simulink library "carnotUIBK_bus"  (R2023b)
settings: Solver=VariableStepAuto  StartTime=0.0  StopTime=10.0  RelTol=1e-3  EnableMultiTasking=on
values from neighbouring files (symbols this model uses):
  A = 7*10*2    (= 140)    [theta_ground_v1.m]    (also in xlswrite1.m = num2cell(data))
  amb_factor = 1    [DOOR.m]    (also in WALL.m; WINDOW.m = 0)
  area = obj.width * obj.height    [DOOR.m]    (also in RES.m = []; ROOM.m = 0; THERMALZONE.m = area + room(kk).area; WALL.m = area - obj.doors(jj).calc_area())
  B = A/(0.5 * P)    (= 8.23529411765)    [theta_ground_v1.m]
  boundary = BOUNDARY()    [BUILDING.m]    (also in WALL.m = '')
  building = obj    [BUILDING.m]    (also in create_building_automatic.m = building.save(); ini_building_automatic.m = building.add_variant_hvac(building.variant_hvac, hvac); load_building_automatic.m = building.save())
  C = zeros(1,length(d)+1)    [CONSTRUCTION.m]    (also in DOOR.m = [0 0 0]; WALL.m = [0 0 0]; WINDOW.m = [0 0 0])
  control = 2    [GAIN.m]    (also in GAINS.m)
  cp = str2num(value)    [CONSTRUCTION.m]
  height = 0    [DOOR.m]    (also in ROOM.m; THERMALZONE.m; WALL.m; WINDOW.m)
  p = [timevec_weather weather(:,12)]    [BOUNDARY.m]    (also in WEATHER.m = 0; init_carnotUIBK.m = cell2mat(carnotUIBKpaths(i,2)))
  rho = str2num(value)    [CONSTRUCTION.m]    (also in theta_ground_v1.m = 2000)
  type = 1    [CONSTRUCTION.m]    (also in GAINS.m = raw_moisture{ii,3}; STRUCTURE.m = 0)
  view_factor = 1    [DOOR.m]    (also in WINDOW.m = 0)
  wall = []    [ROOM.m]
  z = obj.Z    [WALL.m]    (also in theta_ground_v1.m = 0)
  zone = obj.zone(ind)    [THERMALZONE.m]
undefined symbols (not defined in the file or in its folder): const, Dd, get_building, mdot_air, mdot_CO2, mdot_H2O, mdot_VOC, pos, Qdot_C, Qdot_H, Qdot_I_electricity, Qdot_I_light, Qdot_I_person, Qdot_S, Qdot_T_ground, Qdot_T_internal, Qdot_T_neighbour, Qdot_T_opaque, Qdot_T_window, Qdot_V_infiltration, Qdot_V_mech, Qdot_V_window, Qdotc, Qdotr, r_frame, solar_ratio, solar_ratio1, solar_ratio2, Tc, Tr, Ts, Uvalue, wallsurface, window, window_height, window_heigth, window_width, windowsurface, x_CO2, x_H2O, x_VOC
libraries: $bdroot x134, carnot x87, simulink_extras x14, slpidlib x4, simulink x3
(part 6 of 12)

== system carnotUIBK_bus/room_node/1-node/mass blalance ==
  mdot_H2O : Inport
  mdot_CO2 : Inport  Port=2
  mdot_VOC : Inport  Port=3
  AIB : Inport  Port=4
  (1/m^3) : Constant  Value=1/zoneairvolume
  Bus Selector1 : BusSelector  OutputSignals=rho
  m_CO2 : Integrator  InitialCondition=zonestartCO2  LimitOutput=on  LowerSaturationLimit=0
  m_H2O : Integrator  InitialCondition=zonestartWATER  LimitOutput=on  LowerSaturationLimit=0
  m_VOC : Integrator  InitialCondition=zonestartVOC  LimitOutput=on  LowerSaturationLimit=0
  x1 : Product  Inputs=**  InputSameDT=on  SaturateOnIntegerOverflow=on  OutDataTypeStr=Inherit: Same as first input
  x2 : Product  Inputs=**  InputSameDT=on  SaturateOnIntegerOverflow=on  OutDataTypeStr=Inherit: Same as first input
  x3 : Product  Inputs=**  InputSameDT=on  SaturateOnIntegerOverflow=on  OutDataTypeStr=Inherit: Same as first input
  x4 : Product  Inputs=*/  InputSameDT=on  SaturateOnIntegerOverflow=on  OutDataTypeStr=Inherit: Same as first input
  x_H2O : Outport  VectorParamsAs1DForOutWhenUnconnected=off
  x_CO2 : Outport  Port=2  VectorParamsAs1DForOutWhenUnconnected=off
  x_VOC : Outport  Port=3  VectorParamsAs1DForOutWhenUnconnected=off
  wires:
  Bus Selector1/1 -> x4/2  "<rho>"
  AIB/1 -> Bus Selector1/1
  mdot_VOC/1 -> m_VOC/1
  m_CO2/1 -> x2/1
  m_VOC/1 -> x3/1
  x4/1 -> x3/2, x2/2, x1/2
  m_H2O/1 -> x1/1
  x3/1 -> x_VOC/1  "x_VOC"
  (1/m^3)/1 -> x4/1
  x2/1 -> x_CO2/1  "x_CO2"
  x1/1 -> x_H2O/1  "x_H2O"
  mdot_H2O/1 -> m_H2O/1
  mdot_CO2/1 -> m_CO2/1

== system carnotUIBK_bus/room_node/1-node/pressure ==
  mdot_air : Inport
  AIB : Inport  Port=2
  (1/m^3) : Constant  Value=1/zoneairvolume
  Bus Selector1 : BusSelector  OutputSignals=Tc
  Subsystem : Subsystem
  Transfer Fcn (with initial outputs)1 : Subsystem  mask(Transfer Function with Initial Outputs){N=[1], D=[timeconst  1], Y0=zonestartP0, U0=1}
      mask prompts: N "Numerator:"; D "Denominator:"; Y0 "Initial output:"; U0 "Initial input:"
      mask help: Vector expressions for numerator, and denominator. Coefficients are in descending powers of s.
      mask init:
      | [A,B,C,Dd]=tf2ss(N,D);if (isempty(Y0));[m,n]=size(A);X0=zeros(1,m); end; if (isempty(U0));[m,p]=size(B);U0=zeros(1,p);end;X0=getxo(A,B,C,Dd,U0,Y0,0);
      mask Help: Specify the initial output for the transfer function.  An optimization routine attempts to determine the appropriate initial states so that the specified initial output is achieved.  For more details, see the m-file getxo.m
      mask Display: dpoly(N,D,'s')
  m_air : Integrator  InitialCondition=zonestartAIR  LimitOutput=on  LowerSaturationLimit=0
  x : Product  Inputs=***  InputSameDT=on  SaturateOnIntegerOverflow=on  OutDataTypeStr=Inherit: Same as first input
  p : Outport  VectorParamsAs1DForOutWhenUnconnected=off
  wires:
  Transfer Fcn (with initial outputs)1/1(Out1) -> p/1  "p"
  Subsystem/1(R*T ') -> x/2
  (1/m^3)/1 -> x/3
  m_air/1 -> x/1
  AIB/1 -> Bus Selector1/1
  Bus Selector1/1 -> Subsystem/1(T)  "<Tc>"
  x/1 -> Transfer Fcn (with initial outputs)1/1(In1)
  mdot_air/1 -> m_air/1

== system carnotUIBK_bus/room_node/1-node/sensitive_node ==
  note: SENSITIVE node
  Qdotc : Inport
  Qdotr : Inport  Port=2
  Add : Sum
  Integrator : Integrator  InitialCondition=zonestartTEMP
  mcp : Constant  Value=1/mcp
  x3 : Product  Inputs=**  InputSameDT=on  SaturateOnIntegerOverflow=on  OutDataTypeStr=Inherit: Same as first input
  Tc : Outport  VectorParamsAs1DForOutWhenUnconnected=off
  wires:
  x3/1 -> Integrator/1
  Integrator/1 -> Tc/1
  Add/1 -> x3/1
  Qdotc/1 -> Add/2
  Qdotr/1 -> Add/1
  mcp/1 -> x3/2

== system carnotUIBK_bus/room_node/1-node_womass/sensitive_node ==
  note: SENSITIVE node
  Qdotc : Inport
  Qdotr : Inport  Port=2
  Add : Sum
  Integrator : Integrator  InitialCondition=zonestartTEMP
  mcp : Constant  Value=1/mcp
  x3 : Product  Inputs=**  InputSameDT=on  SaturateOnIntegerOverflow=on  OutDataTypeStr=Inherit: Same as first input
  Tc : Outport  VectorParamsAs1DForOutWhenUnconnected=off
  wires:
  x3/1 -> Integrator/1
  Integrator/1 -> Tc/1
  Add/1 -> x3/1
  Qdotc/1 -> Add/2
  Qdotr/1 -> Add/1
  mcp/1 -> x3/2

== system carnotUIBK_bus/room_node/2-node/Sensitive room temperature ==
  note: Sensitive temperature
  Tr : Inport
  Tc : Inport  Port=2
  1-share_c : Gain  Gain=1-share_c  SaturateOnIntegerOverflow=on  OutDataTypeStr=Inherit: Same as input  ParamDataTypeStr=Inherit: Same as input
  Sum : Sum  InputSameDT=on  SaturateOnIntegerOverflow=on  OutDataTypeStr=Inherit: Same as first input
  share_c : Gain  Gain=share_c  SaturateOnIntegerOverflow=on  OutDataTypeStr=Inherit: Same as input  ParamDataTypeStr=Inherit: Same as input
  Ts : Outport  VectorParamsAs1DForOutWhenUnconnected=off
  wires:
  Tr/1 -> 1-share_c/1
  Tc/1 -> share_c/1
  share_c/1 -> Sum/1  "Tc"
  1-share_c/1 -> Sum/2  "Tr"
  Sum/1 -> Ts/1

== system carnotUIBK_bus/room_node/2-node/convective_node ==
  note: CONVECTIVE node
  Qdotc : Inport
  AIB : Inport  Port=2
  (1/m^3) : Constant  Value=1/zoneairvolume
  Bus Selector1 : BusSelector  OutputSignals=rho,cp
  Integrator : Integrator  InitialCondition=zonestartTEMP
  x3 : Product  Inputs=**  InputSameDT=on  SaturateOnIntegerOverflow=on  OutDataTypeStr=Inherit: Same as first input
  x4 : Product  Inputs=*//  InputSameDT=on  SaturateOnIntegerOverflow=on  OutDataTypeStr=Inherit: Same as first input
  Tc : Outport  VectorParamsAs1DForOutWhenUnconnected=off
  wires:
  Bus Selector1/2 -> x4/3  "<cp>"
  Bus Selector1/1 -> x4/2  "<rho>"
  AIB/1 -> Bus Selector1/1
  x3/1 -> Integrator/1
  (1/m^3)/1 -> x4/1
  x4/1 -> x3/2
  Integrator/1 -> Tc/1
  Qdotc/1 -> x3/1

== system carnotUIBK_bus/room_node/2-node/density and capacity ==
  T : Inport
  p : Inport  Port=2
  fluid_type : Inport  Port=3
  fluid_mix : Inport  Port=4
  Add : Sum  Inputs=2
  Constant1 : Constant  Value=10000
  Constant2 : Constant  Value=0.0001
  Divide : Product  Inputs=*/
  K : Constant  Value=273.15
  Product : Product
  Product1 : Product
  Ra : Gain  Gain=287.058
  Rounding Function : Rounding
  Terminator : Terminator
  Terminator1 : Terminator
  Transfer Fcn (with initial outputs) : Subsystem  mask(Transfer Function with Initial Outputs){N=[1], D=[timeconst  1], Y0=1.1893, U0=1}
      mask prompts: N "Numerator:"; D "Denominator:"; Y0 "Initial output:"; U0 "Initial input:"
      mask help: Vector expressions for numerator, and denominator. Coefficients are in descending powers of s.
      mask init:
      | [A,B,C,Dd]=tf2ss(N,D);if (isempty(Y0));[m,n]=size(A);X0=zeros(1,m); end; if (isempty(U0));[m,p]=size(B);U0=zeros(1,p);end;X0=getxo(A,B,C,Dd,U0,Y0,0);
      mask Help: Specify the initial output for the transfer function.  An optimization routine attempts to determine the appropriate initial states so that the specified initial output is achieved.  For more details, see the m-file getxo.m
      mask Display: dpoly(N,D,'s')
  cp_const : Constant  Value=1006.8
  rho : Outport  VectorParamsAs1DForOutWhenUnconnected=off
  cp : Outport  Port=2  VectorParamsAs1DForOutWhenUnconnected=off
  wires:
  cp_const/1 -> cp/1
  Divide/1 -> Transfer Fcn (with initial outputs)/1(In1)
  p/1 -> Divide/1
  fluid_type/1 -> Terminator/1
  fluid_mix/1 -> Terminator1/1
  T/1 -> Add/1
  K/1 -> Add/2
  Add/1 -> Ra/1
  Ra/1 -> Divide/2
  Rounding Function/1 -> Product1/1
  Transfer Fcn (with initial outputs)/1(Out1) -> Product/1
  Product/1 -> Rounding Function/1
  Constant1/1 -> Product/2
  Constant2/1 -> Product1/2
  Product1/1 -> rho/1

== system carnotUIBK_bus/room_node/2-node/mass blalance ==
  mdot_H2O : Inport
  mdot_CO2 : Inport  Port=2
  mdot_VOC : Inport  Port=3
  AIB : Inport  Port=4
  (1/m^3) : Constant  Value=1/zoneairvolume
  Bus Selector1 : BusSelector  OutputSignals=rho
  m_CO2 : Integrator  InitialCondition=zonestartCO2  LimitOutput=on  LowerSaturationLimit=0
  m_H2O : Integrator  InitialCondition=zonestartWATER  LimitOutput=on  LowerSaturationLimit=0
  m_VOC : Integrator  InitialCondition=zonestartVOC  LimitOutput=on  LowerSaturationLimit=0
  x1 : Product  Inputs=**  InputSameDT=on  SaturateOnIntegerOverflow=on  OutDataTypeStr=Inherit: Same as first input
  x2 : Product  Inputs=**  InputSameDT=on  SaturateOnIntegerOverflow=on  OutDataTypeStr=Inherit: Same as first input
  x3 : Product  Inputs=**  InputSameDT=on  SaturateOnIntegerOverflow=on  OutDataTypeStr=Inherit: Same as first input
  x4 : Product  Inputs=*/  InputSameDT=on  SaturateOnIntegerOverflow=on  OutDataTypeStr=Inherit: Same as first input
  x_H2O : Outport  VectorParamsAs1DForOutWhenUnconnected=off
  x_CO2 : Outport  Port=2  VectorParamsAs1DForOutWhenUnconnected=off
  x_VOC : Outport  Port=3  VectorParamsAs1DForOutWhenUnconnected=off
  wires:
  Bus Selector1/1 -> x4/2  "<rho>"
  AIB/1 -> Bus Selector1/1
  mdot_VOC/1 -> m_VOC/1
  m_CO2/1 -> x2/1
  m_VOC/1 -> x3/1
  x4/1 -> x3/2, x2/2, x1/2
  m_H2O/1 -> x1/1
  x3/1 -> x_VOC/1  "x_VOC"
  (1/m^3)/1 -> x4/1
  x2/1 -> x_CO2/1  "x_CO2"
  x1/1 -> x_H2O/1  "x_H2O"
  mdot_H2O/1 -> m_H2O/1
  mdot_CO2/1 -> m_CO2/1

== system carnotUIBK_bus/room_node/2-node/pressure ==
  mdot_air : Inport
  AIB : Inport  Port=2
  (1/m^3) : Constant  Commented=on  Value=1/zoneairvolume
  Bus Selector1 : BusSelector  Commented=on  OutputSignals=Tc
  Subsystem : Subsystem  Commented=on
  Transfer Fcn (with initial outputs)1 : Subsystem  Commented=on  mask(Transfer Function with Initial Outputs){N=[1], D=[timeconst  1], Y0=zonestartP0, U0=1}
      mask prompts: N "Numerator:"; D "Denominator:"; Y0 "Initial output:"; U0 "Initial input:"
      mask help: Vector expressions for numerator, and denominator. Coefficients are in descending powers of s.
      mask init:
      | [A,B,C,Dd]=tf2ss(N,D);if (isempty(Y0));[m,n]=size(A);X0=zeros(1,m); end; if (isempty(U0));[m,p]=size(B);U0=zeros(1,p);end;X0=getxo(A,B,C,Dd,U0,Y0,0);
      mask Help: Specify the initial output for the transfer function.  An optimization routine attempts to determine the appropriate initial states so that the specified initial output is achieved.  For more details, see the m-file getxo.m
      mask Display: dpoly(N,D,'s')
  convert2U32 : DataTypeConversion  Commented=on  OutDataTypeStr=uint32  SaturateOnIntegerOverflow=off  RndMeth=Floor
  convert2double : DataTypeConversion  Commented=on  OutDataTypeStr=double  SaturateOnIntegerOverflow=off  RndMeth=Floor
  m_air : Integrator  Commented=on  InitialCondition=zonestartAIR  LimitOutput=on  LowerSaturationLimit=0
  p0 : Constant  Value=1e5
  x : Product  Commented=on  Inputs=***  InputSameDT=on  SaturateOnIntegerOverflow=on  OutDataTypeStr=Inherit: Same as first input
  p : Outport  VectorParamsAs1DForOutWhenUnconnected=off
  wires:
  Transfer Fcn (with initial outputs)1/1(Out1) -> convert2U32/1  "p"
  Subsystem/1(R*T ') -> x/2
  (1/m^3)/1 -> x/3
  m_air/1 -> x/1
  AIB/1 -> Bus Selector1/1
  Bus Selector1/1 -> Subsystem/1(T)  "<Tc>"
  x/1 -> Transfer Fcn (with initial outputs)1/1(In1)
  mdot_air/1 -> m_air/1
  convert2U32/1 -> convert2double/1
  p0/1 -> p/1

== system carnotUIBK_bus/room_node/2-node/radiative_node ==
  note: RADIATIVE node
  Qdotr : Inport
  Gain : Gain  Gain=1/timeconst
  Integrator : Integrator  InitialCondition=zonestartTEMP
  Tr : Outport  VectorParamsAs1DForOutWhenUnconnected=off
  wires:
  Integrator/1 -> Tr/1
  Qdotr/1 -> Gain/1
  Gain/1 -> Integrator/1

== system carnotUIBK_bus/room_node/2-node_ideal/Sensitive room temperature ==
  note: Sensitive temperature
  Tr : Inport
  Tc : Inport  Port=2
  1-share_c : Gain  Gain=1-share_c  SaturateOnIntegerOverflow=on  OutDataTypeStr=Inherit: Same as input  ParamDataTypeStr=Inherit: Same as input
  Sum : Sum  InputSameDT=on  SaturateOnIntegerOverflow=on  OutDataTypeStr=Inherit: Same as first input
  share_c : Gain  Gain=share_c  SaturateOnIntegerOverflow=on  OutDataTypeStr=Inherit: Same as input  ParamDataTypeStr=Inherit: Same as input
  Ts : Outport  VectorParamsAs1DForOutWhenUnconnected=off
  wires:
  Tr/1 -> 1-share_c/1
  Tc/1 -> share_c/1
  share_c/1 -> Sum/1  "Tc"
  1-share_c/1 -> Sum/2  "Tr"
  Sum/1 -> Ts/1

== system carnotUIBK_bus/room_node/2-node_ideal/mass blalance ==
  mdot_H2O : Inport
  mdot_CO2 : Inport  Port=2
  mdot_VOC : Inport  Port=3
  AIB : Inport  Port=4
  (1/m^3) : Constant  Value=1/zoneairvolume
  Bus Selector1 : BusSelector  OutputSignals=rho
  m_CO2 : Integrator  InitialCondition=zonestartCO2  LimitOutput=on  LowerSaturationLimit=0
  m_H2O : Integrator  InitialCondition=zonestartWATER  LimitOutput=on  LowerSaturationLimit=0
  m_VOC : Integrator  InitialCondition=zonestartVOC  LimitOutput=on  LowerSaturationLimit=0
  x1 : Product  Inputs=**  InputSameDT=on  SaturateOnIntegerOverflow=on  OutDataTypeStr=Inherit: Same as first input
  x2 : Product  Inputs=**  InputSameDT=on  SaturateOnIntegerOverflow=on  OutDataTypeStr=Inherit: Same as first input
  x3 : Product  Inputs=**  InputSameDT=on  SaturateOnIntegerOverflow=on  OutDataTypeStr=Inherit: Same as first input
  x4 : Product  Inputs=*/  InputSameDT=on  SaturateOnIntegerOverflow=on  OutDataTypeStr=Inherit: Same as first input
  x_H2O : Outport  VectorParamsAs1DForOutWhenUnconnected=off
  x_CO2 : Outport  Port=2  VectorParamsAs1DForOutWhenUnconnected=off
  x_VOC : Outport  Port=3  VectorParamsAs1DForOutWhenUnconnected=off
  wires:
  Bus Selector1/1 -> x4/2  "<rho>"
  AIB/1 -> Bus Selector1/1
  mdot_VOC/1 -> m_VOC/1
  m_CO2/1 -> x2/1
  m_VOC/1 -> x3/1
  x4/1 -> x3/2, x2/2, x1/2
  m_H2O/1 -> x1/1
  x3/1 -> x_VOC/1  "x_VOC"
  (1/m^3)/1 -> x4/1
  x2/1 -> x_CO2/1  "x_CO2"
  x1/1 -> x_H2O/1  "x_H2O"
  mdot_H2O/1 -> m_H2O/1
  mdot_CO2/1 -> m_CO2/1

== system carnotUIBK_bus/room_node/2-node_ideal/pressure ==
  mdot_air : Inport
  AIB : Inport  Port=2
  (1/m^3) : Constant  Value=1/zoneairvolume
  Bus Selector1 : BusSelector  OutputSignals=Tc
  Subsystem : Subsystem
  Transfer Fcn (with initial outputs)1 : Subsystem  mask(Transfer Function with Initial Outputs){N=[1], D=[timeconst  1], Y0=zonestartP0, U0=1}
      mask prompts: N "Numerator:"; D "Denominator:"; Y0 "Initial output:"; U0 "Initial input:"
      mask help: Vector expressions for numerator, and denominator. Coefficients are in descending powers of s.
      mask init:
      | [A,B,C,Dd]=tf2ss(N,D);if (isempty(Y0));[m,n]=size(A);X0=zeros(1,m); end; if (isempty(U0));[m,p]=size(B);U0=zeros(1,p);end;X0=getxo(A,B,C,Dd,U0,Y0,0);
      mask Help: Specify the initial output for the transfer function.  An optimization routine attempts to determine the appropriate initial states so that the specified initial output is achieved.  For more details, see the m-file getxo.m
      mask Display: dpoly(N,D,'s')
  m_air : Integrator  InitialCondition=zonestartAIR  LimitOutput=on  LowerSaturationLimit=0
  x : Product  Inputs=***  InputSameDT=on  SaturateOnIntegerOverflow=on  OutDataTypeStr=Inherit: Same as first input
  p : Outport  VectorParamsAs1DForOutWhenUnconnected=off
  wires:
  Transfer Fcn (with initial outputs)1/1(Out1) -> p/1  "p"
  Subsystem/1(R*T ') -> x/2
  (1/m^3)/1 -> x/3
  m_air/1 -> x/1
  AIB/1 -> Bus Selector1/1
  Bus Selector1/1 -> Subsystem/1(T)  "<Tc>"
  x/1 -> Transfer Fcn (with initial outputs)1/1(In1)
  mdot_air/1 -> m_air/1

== system carnotUIBK_bus/room_node/EMPTY/AIB_initialize ==
  Bus Creator2 : BusCreator  Inputs=9
  Constant{,1..8} (9 alike) : Constant  Value=0
  AIB : Outport  VectorParamsAs1DForOutWhenUnconnected=off
  wires:
  Bus Creator2/1 -> AIB/1
  Constant4/1 -> Bus Creator2/5  "x_CO2"
  Constant2/1 -> Bus Creator2/3  "Tr"
  Constant1/1 -> Bus Creator2/2  "Tc"
  Constant6/1 -> Bus Creator2/7  "rho"
  Constant7/1 -> Bus Creator2/8  "cp"
  Constant/1 -> Bus Creator2/1  "Ts"
  Constant8/1 -> Bus Creator2/9  "p"
  Constant3/1 -> Bus Creator2/4  "x_H2O"
  Constant5/1 -> Bus Creator2/6  "x_VOC"

== system carnotUIBK_bus/room_node/EMPTY/Sensitive room temperature ==
  note: Sensitive temperature
  Tr : Inport
  Tc : Inport  Port=2
  1-share_c : Gain  Gain=1-share_c  SaturateOnIntegerOverflow=on  OutDataTypeStr=Inherit: Same as input  ParamDataTypeStr=Inherit: Same as input
  Sum : Sum  InputSameDT=on  SaturateOnIntegerOverflow=on  OutDataTypeStr=Inherit: Same as first input
  share_c : Gain  Gain=share_c  SaturateOnIntegerOverflow=on  OutDataTypeStr=Inherit: Same as input  ParamDataTypeStr=Inherit: Same as input
  Ts : Outport  VectorParamsAs1DForOutWhenUnconnected=off
  wires:
  Tr/1 -> 1-share_c/1
  Tc/1 -> share_c/1
  share_c/1 -> Sum/1  "Tc"
  1-share_c/1 -> Sum/2  "Tr"
  Sum/1 -> Ts/1

== system carnotUIBK_bus/wall_intersection/R-C model/alpha_i1 ==
  Ts : Inport
  AIB : Inport  Port=2
  Qdot sol : Inport  Port=3
  phis : Inport  Port=4
  alpha_i_down : Subsystem  VariantControl=V_i_XXX_XXX_wXXX_hti2  mask(ALFA){}
      mask help:
      | Convective and radiative heat transfer at the INDOOR SURFACE of a VERTICAL OUTER WALL.
      |
      | [AIV] : conditions of zone node,
      | Ts : temperature of wall surface, °C,
      | qdots : specific heat flow into wall construction, W/m^2,
      | [S] : heat and air flow to zone node.
  alpha_i_horizontal : Subsystem  VariantControl=V_i_XXX_XXX_wXXX_hti0  mask(ALFA){}
      mask help:
      | Convective and radiative heat transfer at the INDOOR SURFACE of a VERTICAL OUTER WALL.
      |
      | [AIV] : conditions of zone node,
      | Ts : temperature of wall surface, °C,
      | qdots : specific heat flow into wall construction, W/m^2,
      | [S] : heat and air flow to zone node.
  alpha_i_up : Subsystem  VariantControl=V_i_XXX_XXX_wXXX_hti1  mask(ALFA){}
      mask help:
      | Convective and radiative heat transfer at the INDOOR SURFACE of a VERTICAL OUTER WALL.
      |
      | [AIV] : conditions of zone node,
      | Ts : temperature of wall surface, °C,
      | qdots : specific heat flow into wall construction, W/m^2,
      | [S] : heat and air flow to zone node.
  qdots : Outport  VectorParamsAs1DForOutWhenUnconnected=off
  "[S]" : Outport  Port=2  VectorParamsAs1DForOutWhenUnconnected=off
  alpha_c : Outport  Port=3  VectorParamsAs1DForOutWhenUnconnected=off
  phi_i_1/100 : Outport  Port=4  VectorParamsAs1DForOutWhenUnconnected=off

== system carnotUIBK_bus/wall_intersection/R-C model/alpha_i2 ==
  Ts : Inport
  AIB : Inport  Port=2
  Qdot sol : Inport  Port=3
  phis : Inport  Port=4
  alpha_i_down : Subsystem  VariantControl=V_i_XXX_XXX_wXXX_hti2  mask(ALFA){}
      mask help:
      | Convective and radiative heat transfer at the INDOOR SURFACE of a VERTICAL OUTER WALL.
      |
      | [AIV] : conditions of zone node,
      | Ts : temperature of wall surface, °C,
      | qdots : specific heat flow into wall construction, W/m^2,
      | [S] : heat and air flow to zone node.
  alpha_i_horizontal : Subsystem  VariantControl=V_i_XXX_XXX_wXXX_hti0  mask(ALFA){}
      mask help:
      | Convective and radiative heat transfer at the INDOOR SURFACE of a VERTICAL OUTER WALL.
      |
      | [AIV] : conditions of zone node,
      | Ts : temperature of wall surface, °C,
      | qdots : specific heat flow into wall construction, W/m^2,
      | [S] : heat and air flow to zone node.
  alpha_i_up : Subsystem  VariantControl=V_i_XXX_XXX_wXXX_hti1  mask(ALFA){}
      mask help:
      | Convective and radiative heat transfer at the INDOOR SURFACE of a VERTICAL OUTER WALL.
      |
      | [AIV] : conditions of zone node,
      | Ts : temperature of wall surface, °C,
      | qdots : specific heat flow into wall construction, W/m^2,
      | [S] : heat and air flow to zone node.
  qdots : Outport  VectorParamsAs1DForOutWhenUnconnected=off
  "[S]" : Outport  Port=2  VectorParamsAs1DForOutWhenUnconnected=off
  alpha_c : Outport  Port=3  VectorParamsAs1DForOutWhenUnconnected=off
  phi_i_1/100 : Outport  Port=4  VectorParamsAs1DForOutWhenUnconnected=off

== system carnotUIBK_bus/wall_intersection/UA/Rsi ==
  down : Subsystem  VariantControl=V_i_XXX_XXX_wXXX_hti2
  horizontal : Subsystem  VariantControl=V_i_XXX_XXX_wXXX_hti0
  up : Subsystem  VariantControl=V_i_XXX_XXX_wXXX_hti1
  Rsi : Outport  VectorParamsAs1DForOutWhenUnconnected=off

== system carnotUIBK_bus/wall_intersection/hygrothermal model/alpha_i1 ==
  Ts : Inport
  AIB : Inport  Port=2
  Qdot sol : Inport  Port=3
  phis : Inport  Port=4
  alpha_i_down : Subsystem  VariantControl=V_i_XXX_XXX_wXXX_hti2  mask(ALFA){}
      mask help:
      | Convective and radiative heat transfer at the INDOOR SURFACE of a VERTICAL OUTER WALL.
      |
      | [AIV] : conditions of zone node,
      | Ts : temperature of wall surface, °C,
      | qdots : specific heat flow into wall construction, W/m^2,
      | [S] : heat and air flow to zone node.
  alpha_i_horizontal : Subsystem  VariantControl=V_i_XXX_XXX_wXXX_hti0  mask(ALFA){}
      mask help:
      | Convective and radiative heat transfer at the INDOOR SURFACE of a VERTICAL OUTER WALL.
      |
      | [AIV] : conditions of zone node,
      | Ts : temperature of wall surface, °C,
      | qdots : specific heat flow into wall construction, W/m^2,
      | [S] : heat and air flow to zone node.
  alpha_i_up : Subsystem  VariantControl=V_i_XXX_XXX_wXXX_hti1  mask(ALFA){}
      mask help:
      | Convective and radiative heat transfer at the INDOOR SURFACE of a VERTICAL OUTER WALL.
      |
      | [AIV] : conditions of zone node,
      | Ts : temperature of wall surface, °C,
      | qdots : specific heat flow into wall construction, W/m^2,
      | [S] : heat and air flow to zone node.
  qdots : Outport  VectorParamsAs1DForOutWhenUnconnected=off
  "[S]" : Outport  Port=2  VectorParamsAs1DForOutWhenUnconnected=off
  alpha_c : Outport  Port=3  VectorParamsAs1DForOutWhenUnconnected=off
  phi_i_1/100 : Outport  Port=4  VectorParamsAs1DForOutWhenUnconnected=off

== system carnotUIBK_bus/wall_intersection/hygrothermal model/alpha_i2 ==
  Ts : Inport
  AIB : Inport  Port=2
  Qdot sol : Inport  Port=3
  phis : Inport  Port=4
  alpha_i_down : Subsystem  VariantControl=V_i_XXX_XXX_wXXX_hti2  mask(ALFA){}
      mask help:
      | Convective and radiative heat transfer at the INDOOR SURFACE of a VERTICAL OUTER WALL.
      |
      | [AIV] : conditions of zone node,
      | Ts : temperature of wall surface, °C,
      | qdots : specific heat flow into wall construction, W/m^2,
      | [S] : heat and air flow to zone node.
  alpha_i_horizontal : Subsystem  VariantControl=V_i_XXX_XXX_wXXX_hti0  mask(ALFA){}
      mask help:
      | Convective and radiative heat transfer at the INDOOR SURFACE of a VERTICAL OUTER WALL.
      |
      | [AIV] : conditions of zone node,
      | Ts : temperature of wall surface, °C,
      | qdots : specific heat flow into wall construction, W/m^2,
      | [S] : heat and air flow to zone node.
  alpha_i_up : Subsystem  VariantControl=V_i_XXX_XXX_wXXX_hti1  mask(ALFA){}
      mask help:
      | Convective and radiative heat transfer at the INDOOR SURFACE of a VERTICAL OUTER WALL.
      |
      | [AIV] : conditions of zone node,
      | Ts : temperature of wall surface, °C,
      | qdots : specific heat flow into wall construction, W/m^2,
      | [S] : heat and air flow to zone node.
  qdots : Outport  VectorParamsAs1DForOutWhenUnconnected=off
  "[S]" : Outport  Port=2  VectorParamsAs1DForOutWhenUnconnected=off
  alpha_c : Outport  Port=3  VectorParamsAs1DForOutWhenUnconnected=off
  phi_i_1/100 : Outport  Port=4  VectorParamsAs1DForOutWhenUnconnected=off

== system carnotUIBK_bus/wall_zone/R-C model/alpha_e ==
  WDB : Inport
  GDB : Inport  Port=2
  NDB : Inport  Port=3
  AIB : Inport  Port=4
  Ts : Inport  Port=5
  Qdot_sol : Inport  Port=6
  phis : Inport  Port=7
  alpha_e_AMBIENT : Subsystem  VariantControl=V_zXXX_wXXX_hte0  mask(ALFA){}
      mask help:
      | Convective and radiative HEAT TRANSFER at the WEATHER EXPOSED SURFACE of an OUTER WALL.
      |
      | [W*] : modified weather data, adapted to height over ground,
      | Ts : temperature of outdoor wall surface, °C,
      | qdots : specific heat flow into wall / window construction, W/m^2.
  alpha_e_GROUND : Subsystem  VariantControl=V_zXXX_wXXX_hte1  mask(ALFA){}
      mask help:
      | Convective and radiative HEAT TRANSFER at the WEATHER EXPOSED SURFACE of an OUTER WALL.
      |
      | [W*] : modified weather data, adapted to height over ground,
      | Ts : temperature of outdoor wall surface, °C,
      | qdots : specific heat flow into wall / window construction, W/m^2.
  alpha_e_INTERNAL : Subsystem  VariantControl=V_zXXX_wXXX_hte2  mask(ALFA){}
      mask help:
      | Convective and radiative HEAT TRANSFER at the WEATHER EXPOSED SURFACE of an OUTER WALL.
      |
      | [W*] : modified weather data, adapted to height over ground,
      | Ts : temperature of outdoor wall surface, °C,
      | qdots : specific heat flow into wall / window construction, W/m^2.
  alpha_e_NEIGHBOUR : Subsystem  VariantControl=V_zXXX_wXXX_hte3  mask(ALFA){}
      mask help:
      | Convective and radiative HEAT TRANSFER at the WEATHER EXPOSED SURFACE of an OUTER WALL.
      |
      | [W*] : modified weather data, adapted to height over ground,
      | Ts : temperature of outdoor wall surface, °C,
      | qdots : specific heat flow into wall / window construction, W/m^2.
  qdots : Outport  VectorParamsAs1DForOutWhenUnconnected=off
  "[S]" : Outport  Port=2  VectorParamsAs1DForOutWhenUnconnected=off
  alpha_c : Outport  Port=3  VectorParamsAs1DForOutWhenUnconnected=off
  phi_e_1/100 : Outport  Port=4  VectorParamsAs1DForOutWhenUnconnected=off
  theta_e : Outport  Port=5  VectorParamsAs1DForOutWhenUnconnected=off

== system carnotUIBK_bus/wall_zone/R-C model/alpha_i ==
  Ts : Inport
  AIB : Inport  Port=2
  Qdot sol : Inport  Port=3
  phis : Inport  Port=4
  alpha_i_down : Subsystem  VariantControl=V_zXXX_wXXX_hti2  mask(ALFA){}
      mask help:
      | Convective and radiative heat transfer at the INDOOR SURFACE of a VERTICAL OUTER WALL.
      |
      | [AIV] : conditions of zone node,
      | Ts : temperature of wall surface, °C,
      | qdots : specific heat flow into wall construction, W/m^2,
      | [S] : heat and air flow to zone node.
  alpha_i_horizontal : Subsystem  VariantControl=V_zXXX_wXXX_hti0  mask(ALFA){}
      mask help:
      | Convective and radiative heat transfer at the INDOOR SURFACE of a VERTICAL OUTER WALL.
      |
      | [AIV] : conditions of zone node,
      | Ts : temperature of wall surface, °C,
      | qdots : specific heat flow into wall construction, W/m^2,
      | [S] : heat and air flow to zone node.
  alpha_i_up : Subsystem  VariantControl=V_zXXX_wXXX_hti1  mask(ALFA){}
      mask help:
      | Convective and radiative heat transfer at the INDOOR SURFACE of a VERTICAL OUTER WALL.
      |
      | [AIV] : conditions of zone node,
      | Ts : temperature of wall surface, °C,
      | qdots : specific heat flow into wall construction, W/m^2,
      | [S] : heat and air flow to zone node.
  qdots : Outport  VectorParamsAs1DForOutWhenUnconnected=off
  "[S]" : Outport  Port=2  VectorParamsAs1DForOutWhenUnconnected=off
  alpha_c : Outport  Port=3  VectorParamsAs1DForOutWhenUnconnected=off
  phi_i_1/100 : Outport  Port=4  VectorParamsAs1DForOutWhenUnconnected=off

== system carnotUIBK_bus/wall_zone/UA/Rse ==
  WDB : Inport
  GDB : Inport  Port=2
  NDB : Inport  Port=3
  AIB : Inport  Port=4
  Qdot_sol : Inport  Port=5
  Qdot_in : Inport  Port=6
  R : Inport  Port=7
  Rsi : Inport  Port=8
  AMBIENT : Subsystem  VariantControl=V_zXXX_wXXX_hte0
  GROUND : Subsystem  VariantControl=V_zXXX_wXXX_hte1
  INTERNAL : Subsystem  VariantControl=V_zXXX_wXXX_hte2
  NEIGHBOUR : Subsystem  VariantControl=V_zXXX_wXXX_hte3
  "[S]" : Outport  VectorParamsAs1DForOutWhenUnconnected=off

== system carnotUIBK_bus/wall_zone/UA/Rsi ==
  down : Subsystem  VariantControl=V_zXXX_wXXX_hti2
  horizontal : Subsystem  VariantControl=V_zXXX_wXXX_hti0
  up : Subsystem  VariantControl=V_zXXX_wXXX_hti1
  Rsi : Outport  VectorParamsAs1DForOutWhenUnconnected=off

== system carnotUIBK_bus/wall_zone/hygrothermal model/alpha_e ==
  WDB : Inport
  GDB : Inport  Port=2
  NDB : Inport  Port=3
  AIB : Inport  Port=4
  Ts : Inport  Port=5
  Qdot_sol : Inport  Port=6
  phis : Inport  Port=7
  alpha_e_AMBIENT : Subsystem  VariantControl=V_zXXX_wXXX_hte0  mask(ALFA){}
      mask help:
      | Convective and radiative HEAT TRANSFER at the WEATHER EXPOSED SURFACE of an OUTER WALL.
      |
      | [W*] : modified weather data, adapted to height over ground,
      | Ts : temperature of outdoor wall surface, °C,
      | qdots : specific heat flow into wall / window construction, W/m^2.
  alpha_e_GROUND : Subsystem  VariantControl=V_zXXX_wXXX_hte1  mask(ALFA){}
      mask help:
      | Convective and radiative HEAT TRANSFER at the WEATHER EXPOSED SURFACE of an OUTER WALL.
      |
      | [W*] : modified weather data, adapted to height over ground,
      | Ts : temperature of outdoor wall surface, °C,
      | qdots : specific heat flow into wall / window construction, W/m^2.
  alpha_e_INTERNAL : Subsystem  VariantControl=V_zXXX_wXXX_hte2  mask(ALFA){}
      mask help:
      | Convective and radiative HEAT TRANSFER at the WEATHER EXPOSED SURFACE of an OUTER WALL.
      |
      | [W*] : modified weather data, adapted to height over ground,
      | Ts : temperature of outdoor wall surface, °C,
      | qdots : specific heat flow into wall / window construction, W/m^2.
  alpha_e_NEIGHBOUR : Subsystem  VariantControl=V_zXXX_wXXX_hte3  mask(ALFA){}
      mask help:
      | Convective and radiative HEAT TRANSFER at the WEATHER EXPOSED SURFACE of an OUTER WALL.
      |
      | [W*] : modified weather data, adapted to height over ground,
      | Ts : temperature of outdoor wall surface, °C,
      | qdots : specific heat flow into wall / window construction, W/m^2.
  qdots : Outport  VectorParamsAs1DForOutWhenUnconnected=off
  "[S]" : Outport  Port=2  VectorParamsAs1DForOutWhenUnconnected=off
  alpha_c : Outport  Port=3  VectorParamsAs1DForOutWhenUnconnected=off
  phi_e_1/100 : Outport  Port=4  VectorParamsAs1DForOutWhenUnconnected=off
  theta_e : Outport  Port=5  VectorParamsAs1DForOutWhenUnconnected=off

== system carnotUIBK_bus/wall_zone/hygrothermal model/alpha_i ==
  Ts : Inport
  AIB : Inport  Port=2
  Qdot sol : Inport  Port=3
  phis : Inport  Port=4
  alpha_i_down : Subsystem  VariantControl=V_zXXX_wXXX_hti2  mask(ALFA){}
      mask help:
      | Convective and radiative heat transfer at the INDOOR SURFACE of a VERTICAL OUTER WALL.
      |
      | [AIV] : conditions of zone node,
      | Ts : temperature of wall surface, °C,
      | qdots : specific heat flow into wall construction, W/m^2,
      | [S] : heat and air flow to zone node.
  alpha_i_horizontal : Subsystem  VariantControl=V_zXXX_wXXX_hti0  mask(ALFA){}
      mask help:
      | Convective and radiative heat transfer at the INDOOR SURFACE of a VERTICAL OUTER WALL.
      |
      | [AIV] : conditions of zone node,
      | Ts : temperature of wall surface, °C,
      | qdots : specific heat flow into wall construction, W/m^2,
      | [S] : heat and air flow to zone node.
  alpha_i_up : Subsystem  VariantControl=V_zXXX_wXXX_hti1  mask(ALFA){}
      mask help:
      | Convective and radiative heat transfer at the INDOOR SURFACE of a VERTICAL OUTER WALL.
      |
      | [AIV] : conditions of zone node,
      | Ts : temperature of wall surface, °C,
      | qdots : specific heat flow into wall construction, W/m^2,
      | [S] : heat and air flow to zone node.
  qdots : Outport  VectorParamsAs1DForOutWhenUnconnected=off
  "[S]" : Outport  Port=2  VectorParamsAs1DForOutWhenUnconnected=off
  alpha_c : Outport  Port=3  VectorParamsAs1DForOutWhenUnconnected=off
  phi_i_1/100 : Outport  Port=4  VectorParamsAs1DForOutWhenUnconnected=off

== system carnotUIBK_bus/window/window_CARNOT/alfa_window_in ==
  note: (W/m^2)
  note: CONVENTION:
      | Qdot > 0 and qdots < 0, if Ts > T (heat flows from wall surface to room node),
      | Qdot < 0 and qdots > 0, if Ts < T (heat flows from room node to wall surface).
  note: s: surface
      | c: convective
      | r: radiative
  note: WINDOW = FRAME + GLASS
  note: (W/m^2)
  note: Convective and radiative heat transfer at the INDOOR SURFACE OF A VERTICAL WINDOW
      | with 1-4 layers (each 3 ... 8 mm thick)
  note: (°C)
  Ts2 : Inport
  "[sun_t]" : Inport  Port=2
  "[AIV]" : Inport  Port=3
  Bus Assignment2 : BusAssignment  AssignedSignals=Qdotc,Qdotr,Qdot_S
  Demux : Demux  Outputs=[1 1 1 6]
      settings: DisplayOption=none
  Demux1 : Demux  Outputs=[1 2]
      settings: DisplayOption=none
  Irradiation into room : Subsystem
  Product5 : Product  InputSameDT=on  SaturateOnIntegerOverflow=on  OutDataTypeStr=Inherit: Same as first input
  S_initialize : $bdroot/general/S_initialize  SystemSampleTime=-1  VariantActivationTime=update diagram  AllowFlexibleInterface=on  Latency=0  AutoFrameSizeCalculation=off
  Sum : Sum  Inputs=-+  InputSameDT=on  SaturateOnIntegerOverflow=on  OutDataTypeStr=Inherit: Same as first input
  Sum1 : Sum  Inputs=+-  InputSameDT=on  SaturateOnIntegerOverflow=on  OutDataTypeStr=Inherit: Same as first input
  Sum2 : Sum  Inputs=--  InputSameDT=on  SaturateOnIntegerOverflow=on  OutDataTypeStr=Inherit: Same as first input
  Terminator : Terminator
  Terminator1 : Terminator
  emission_in : Gain  Gain=emission_in  SaturateOnIntegerOverflow=on  OutDataTypeStr=Inherit: Same as input  ParamDataTypeStr=Inherit: Same as input
  surface of window glass : Gain  Gain=(1-frame)*wallsurface  SaturateOnIntegerOverflow=on  OutDataTypeStr=Inherit: Same as input  ParamDataTypeStr=Inherit: Same as input
  surface of window1 : Gain  Gain=wallsurface  SaturateOnIntegerOverflow=on  OutDataTypeStr=Inherit: Same as input  ParamDataTypeStr=Inherit: Same as input
  surface of window2 : Gain  Gain=wallsurface  SaturateOnIntegerOverflow=on  OutDataTypeStr=Inherit: Same as input  ParamDataTypeStr=Inherit: Same as input
  transmission coefficient 1-2-3-4-layer(s) : Subsystem
  u_convection : Gain  Gain=2.5  SaturateOnIntegerOverflow=on  OutDataTypeStr=Inherit: Same as input  ParamDataTypeStr=Inherit: Same as input
  u_rad : Constant  Value=5.6
  u_rad1 : Constant  Value=zeros(numlayer,1)
  qdots2 : Outport  InitialOutput=0  VectorParamsAs1DForOutWhenUnconnected=off
  qdot_abs : Outport  Port=2  InitialOutput=0  VectorParamsAs1DForOutWhenUnconnected=off
  "[S]" : Outport  Port=3  InitialOutput=0  VectorParamsAs1DForOutWhenUnconnected=off
  wires:
  Sum2/1 -> qdots2/1
  Demux/4 -> Terminator1/1
  "[AIV]"/1 -> Demux/1
  Demux/1 -> Terminator/1
  emission_in/1 -> Product5/1
  Sum1/1 -> Product5/2  "dTr"
  u_rad/1 -> emission_in/1
  Ts2/1 -> Sum/2, Sum1/1  "Ts"
  Product5/1 -> Sum2/2, surface of window2/1  "qdotr"
  u_convection/1 -> surface of window1/1, Sum2/1  "qdotc"
  Irradiation into room/1(qdot_sol) -> surface of window glass/1  "qdot_sol (>= 0)"
  Demux1/1 -> transmission coefficient 1-2-3-4-layer(s)/1(teta)  "teta"
  "[sun_t]"/1 -> Demux1/1
  Demux/2 -> Sum/1  "Tc"
  u_rad1/1 -> qdot_abs/1
  Sum/1 -> u_convection/1  "dTc"
  Demux/3 -> Sum1/2  "Tr"
  Demux1/2 -> Irradiation into room/1("[I_t]")  "[I_t]"
  transmission coefficient 1-2-3-4-layer(s)/1("[tau]") -> Irradiation into room/2("[tau]")
  surface of window glass/1 -> Bus Assignment2/4  "Qdot_sol"
  S_initialize/1 -> Bus Assignment2/1
  Bus Assignment2/1 -> "[S]"/1
  surface of window1/1 -> Bus Assignment2/2  "[Qdotc, Qdotr]"
  surface of window2/1 -> Bus Assignment2/3  "[Qdotc, Qdotr]"

== system carnotUIBK_bus/window/window_CARNOT/alfa_window_out ==
  note: WINDOW = FRAME + GLASS
  note: Convective and radiative heat transfer at the OUTDOOR SURFACE OF A VERTICAL WINDOW
  note: modified
      | weatherdata
  note: s: surface
      | c: convective
      | r: radiative
      | h: in height
      | t: tilted surface
  note: CONVENTION:
      | qdots < 0, if Ts > T, heat flows from window surface (resp. room node) to ambition,
      | qdots > 0, if Ts < T, heat flows from ambition to window surface (resp. room node).
  WDB : Inport
  g : Inport  Port=2
  Ts1 : Inport  Port=3
  Bus Assignment2 : BusAssignment  AssignedSignals=Qdot_T_window
  Bus Selector : BusSelector  OutputSignals=Temperature_Ambient,Temperature_Sky_Radiation,Wind_Speed
  Bus Selector1 : BusSelector  OutputSignals=Incidence_Angle_sun,Solar_Radiation_direct_surface,Solar_Radiation_diffuse_surface
  Mux1 : Mux  Inputs=2
  Mux2 : Mux  Inputs=2
  Product6 : Product  InputSameDT=on  SaturateOnIntegerOverflow=on  OutDataTypeStr=Inherit: Same as first input
  Product7 : Product  InputSameDT=on  SaturateOnIntegerOverflow=on  OutDataTypeStr=Inherit: Same as first input
  Radiation_on_Inclined_Surface : carnot/Weather/Radiation_on_Inclined_Surface  sky=Perez 1990  reflect=0.2
      settings: SourceProductName=Carnot
  S_initialize : $bdroot/general/S_initialize  SystemSampleTime=-1  VariantActivationTime=update diagram  AllowFlexibleInterface=on  Latency=0  AutoFrameSizeCalculation=off
  Sum : Sum  Inputs=+-  InputSameDT=on  SaturateOnIntegerOverflow=on  OutDataTypeStr=Inherit: Same as first input
  Sum2 : Sum  Inputs=+++  InputSameDT=on  SaturateOnIntegerOverflow=on  OutDataTypeStr=Inherit: Same as first input
  Sum3 : Sum  InputSameDT=on  SaturateOnIntegerOverflow=on  OutDataTypeStr=Inherit: Same as first input
  absorption_out * frame : Gain  Gain=absorption_out * frame  SaturateOnIntegerOverflow=on  OutDataTypeStr=Inherit: Same as input  ParamDataTypeStr=Inherit: Same as input
  alfa : Fcn  Expr=3*u(1)+2.8
  position : Constant  Value=pos
  qp rad : Subsystem
  surface of window : Gain  Gain=windowsurface  SaturateOnIntegerOverflow=on  OutDataTypeStr=Inherit: Same as input  ParamDataTypeStr=Inherit: Same as input
  "[sun_t]" : Outport  InitialOutput=0  VectorParamsAs1DForOutWhenUnconnected=off
  qdots1 : Outport  Port=2  InitialOutput=0  VectorParamsAs1DForOutWhenUnconnected=off
  "[S]" : Outport  Port=3  InitialOutput=0  VectorParamsAs1DForOutWhenUnconnected=off
  wires:
  Radiation_on_Inclined_Surface/1 -> Bus Selector1/1
  position/1 -> Radiation_on_Inclined_Surface/2
  Product7/1 -> Sum2/1  "qdot,conv"
  alfa/1 -> Product7/2  "alfa"
  qp rad/1(qprad) -> Sum2/2  "qdotr"
  Ts1/1 -> qp rad/2(Tw), Sum/2  "Ts (outer wall surface)"
  Mux1/1 -> "[sun_t]"/1
  Bus Selector1/2 -> Mux2/1, Sum3/1  "<Solar_Radiation_direct_surface>"
  absorption_out * frame/1 -> Sum2/3
  g/1 -> Product6/2
  Sum2/1 -> surface of window/1, qdots1/1
  Sum3/1 -> absorption_out * frame/1
  Bus Selector1/1 -> Mux1/1  "<Incidence_Angle_sun>"
  WDB/1 -> Radiation_on_Inclined_Surface/1, Bus Selector/1
  Sum/1 -> Product7/1  "dTc"
  Product6/1 -> Mux1/2
  Mux2/1 -> Product6/1
  Bus Selector1/3 -> Mux2/2, Sum3/2  "<Solar_Radiation_diffuse_surface>"
  Bus Selector/1 -> qp rad/1(Ta), Sum/1  "<Temperature_Ambient>"
  Bus Selector/2 -> qp rad/3(Tsky)  "<Temperature_Sky_Radiation>"
  Bus Selector/3 -> alfa/1  "<Wind_Speed>"
  S_initialize/1 -> Bus Assignment2/1
  surface of window/1 -> Bus Assignment2/2
  Bus Assignment2/1 -> "[S]"/1

== system carnotUIBK_bus/window/window_TF/alfa_window_in ==
  note: Convective and radiative heat transfer at the INDOOR SURFACE OF A VERTICAL WINDOW
      | with 1-4 layers (each 3 ... 8 mm thick)
  note: WINDOW = FRAME + GLASS
  note: s: surface
      | c: convective
      | r: radiative
  note: CONVENTION:
      | Qdot > 0 and qdots < 0, if Ts > T (heat flows from wall surface to room node),
      | Qdot < 0 and qdots > 0, if Ts < T (heat flows from room node to wall surface).
  note: (W/m^2)
  Ts2 : Inport
  "[sun_t]" : Inport  Port=2
  "[AIV]" : Inport  Port=3
  WDB : Inport  Port=4
  control : Inport  Port=5
  Bus Assignment2 : BusAssignment  AssignedSignals=Qdotc,Qdotr,Qdot_S
  Bus Selector : BusSelector  OutputSignals=Tc,Tr
  Fcn : Fcn  Expr=1.6*(abs(u(1)-u(2)))^0.3
  Fcn1 : Fcn  Expr=(273.15+u(1))^4-(273.15+u(2))^4
  Mux2 : Mux  Inputs=2
  Mux3 : Mux  Inputs=2
  Product : Product  InputSameDT=on  RndMeth=Zero  SaturateOnIntegerOverflow=on  OutDataTypeStr=Inherit: Same as first input
  Product1 : Product  InputSameDT=on  RndMeth=Zero  SaturateOnIntegerOverflow=on  OutDataTypeStr=Inherit: Same as first input
  S_initialize : $bdroot/general/S_initialize  SystemSampleTime=-1  VariantActivationTime=update diagram  AllowFlexibleInterface=on  Latency=0  AutoFrameSizeCalculation=off
  Sum : Sum  Inputs=+-  InputSameDT=on  SaturateOnIntegerOverflow=on  OutDataTypeStr=Inherit: Same as first input
  Sum2 : Sum  Inputs=--+  InputSameDT=on  SaturateOnIntegerOverflow=on  OutDataTypeStr=Inherit: Same as first input
  emission_in : Gain  Gain=emission_in  SaturateOnIntegerOverflow=on  OutDataTypeStr=Inherit: Same as input  ParamDataTypeStr=Inherit: Same as input
  glass ratio : Gain  Gain=(1-frame)  SaturateOnIntegerOverflow=on  OutDataTypeStr=Inherit: Same as input  ParamDataTypeStr=Inherit: Same as input
  sigma : Constant  Value=5.67e-8
  surface of window glass : Gain  Gain=(1-frame)*windowsurface  SaturateOnIntegerOverflow=on  OutDataTypeStr=Inherit: Same as input  ParamDataTypeStr=Inherit: Same as input
  surface of window1 : Gain  Gain=windowsurface  SaturateOnIntegerOverflow=on  OutDataTypeStr=Inherit: Same as input  ParamDataTypeStr=Inherit: Same as input
  surface of window2 : Gain  Gain=windowsurface  SaturateOnIntegerOverflow=on  OutDataTypeStr=Inherit: Same as input  ParamDataTypeStr=Inherit: Same as input
  transmission_absorption : Subsystem
  view_factor : Gain  Gain=view_factor  SaturateOnIntegerOverflow=on  OutDataTypeStr=Inherit: Same as input  ParamDataTypeStr=Inherit: Same as input
  qdots2 : Outport  VectorParamsAs1DForOutWhenUnconnected=off
  "[S]" : Outport  Port=2  VectorParamsAs1DForOutWhenUnconnected=off
  wires:
  control/1 -> transmission_absorption/3(control)
  WDB/1 -> transmission_absorption/2(WDB)
  transmission_absorption/1(qdot_abs) -> glass ratio/1  "qabs"
  transmission_absorption/2(qdot_sol) -> surface of window glass/1  "qdot_sol (>=0)"
  surface of window glass/1 -> Bus Assignment2/4  "Qdot_sol"
  "[sun_t]"/1 -> transmission_absorption/1(sun_t)
  Product/1 -> Sum2/2, surface of window2/1  "qdotr"
  Sum2/1 -> qdots2/1
  emission_in/1 -> view_factor/1
  sigma/1 -> emission_in/1
  Fcn1/1 -> Product/2
  view_factor/1 -> Product/1
  "[AIV]"/1 -> Bus Selector/1
  Mux3/1 -> Fcn1/1
  Bus Selector/2 -> Mux3/2  "<Tr>"
  Fcn/1 -> Product1/2  "hc"
  Mux2/1 -> Fcn/1
  Sum/1 -> Product1/1  "dTc"
  Ts2/1 -> Sum/1, Mux2/1, Mux3/1  "Ts"
  Bus Selector/1 -> Sum/2, Mux2/2  "<Tc>"
  Product1/1 -> surface of window1/1, Sum2/1  "qdotc"
  glass ratio/1 -> Sum2/3  "Qdot_sol"
  S_initialize/1 -> Bus Assignment2/1
  surface of window1/1 -> Bus Assignment2/2  "Qdotc"
  surface of window2/1 -> Bus Assignment2/3  "Qdotr"
  Bus Assignment2/1 -> "[S]"/1

== system carnotUIBK_bus/window/window_TF/alfa_window_out ==
  note: WINDOW = FRAME + GLASS
  note: Convective and radiative heat transfer at the OUTDOOR SURFACE OF A VERTICAL WINDOW
  note: modified
      | weatherdata
  note: s: surface
      | c: convective
      | r: radiative
      | h: in height
      | t: tilted surface
  note: CONVENTION:
      | qdots < 0, if Ts > T, heat flows from window surface (resp. room node) to ambition,
      | qdots > 0, if Ts < T, heat flows from ambition to window surface (resp. room node).
  WDB : Inport
  g : Inport  Port=2
  Ts1 : Inport  Port=3
  Bus Assignment2 : BusAssignment  AssignedSignals=Qdot_T_window
  Bus Selector : BusSelector  OutputSignals=Temperature_Ambient,Temperature_Sky_Radiation,Wind_Speed
  Bus Selector1 : BusSelector  OutputSignals=Incidence_Angle_sun,Solar_Radiation_direct_surface,Solar_Radiation_diffuse_surface
  Mux1 : Mux  Inputs=2
  Mux2 : Mux  Inputs=2
  Product6 : Product  InputSameDT=on  SaturateOnIntegerOverflow=on  OutDataTypeStr=Inherit: Same as first input
  Product7 : Product  InputSameDT=on  SaturateOnIntegerOverflow=on  OutDataTypeStr=Inherit: Same as first input
  Radiation_on_Inclined_Surface : carnot/Weather/Radiation_on_Inclined_Surface  sky=Perez 1990  reflect=0.2
      settings: SourceProductName=Carnot
  S_initialize : $bdroot/general/S_initialize  SystemSampleTime=-1  VariantActivationTime=update diagram  AllowFlexibleInterface=on  Latency=0  AutoFrameSizeCalculation=off
  Sum : Sum  Inputs=+-  InputSameDT=on  SaturateOnIntegerOverflow=on  OutDataTypeStr=Inherit: Same as first input
  Sum2 : Sum  Inputs=+++  InputSameDT=on  SaturateOnIntegerOverflow=on  OutDataTypeStr=Inherit: Same as first input
  Sum3 : Sum  InputSameDT=on  SaturateOnIntegerOverflow=on  OutDataTypeStr=Inherit: Same as first input
  absorption_out * frame : Gain  Gain=absorption_out * frame  SaturateOnIntegerOverflow=on  OutDataTypeStr=Inherit: Same as input  ParamDataTypeStr=Inherit: Same as input
  alfa : Fcn  Expr=3*u(1)+2.8
  position : Constant  Value=pos
  qp rad : Subsystem
  surface of window : Gain  Gain=windowsurface  SaturateOnIntegerOverflow=on  OutDataTypeStr=Inherit: Same as input  ParamDataTypeStr=Inherit: Same as input
  "[sun_t]" : Outport  InitialOutput=0  VectorParamsAs1DForOutWhenUnconnected=off
  qdots1 : Outport  Port=2  InitialOutput=0  VectorParamsAs1DForOutWhenUnconnected=off
  "[S]" : Outport  Port=3  InitialOutput=0  VectorParamsAs1DForOutWhenUnconnected=off
  wires:
  Radiation_on_Inclined_Surface/1 -> Bus Selector1/1
  position/1 -> Radiation_on_Inclined_Surface/2
  Product7/1 -> Sum2/1  "qdot,conv"
  alfa/1 -> Product7/2  "alfa"
  qp rad/1(qprad) -> Sum2/2  "qdotr"
  Ts1/1 -> qp rad/2(Tw), Sum/2  "Ts (outer wall surface)"
  Mux1/1 -> "[sun_t]"/1
  Bus Selector1/2 -> Mux2/1, Sum3/1  "<Solar_Radiation_direct_surface>"
  absorption_out * frame/1 -> Sum2/3
  g/1 -> Product6/2
  Sum2/1 -> surface of window/1, qdots1/1
  Sum3/1 -> absorption_out * frame/1
  Bus Selector1/1 -> Mux1/1  "<Incidence_Angle_sun>"
  WDB/1 -> Radiation_on_Inclined_Surface/1, Bus Selector/1
  Sum/1 -> Product7/1  "dTc"
  Product6/1 -> Mux1/2
  Mux2/1 -> Product6/1
  Bus Selector1/3 -> Mux2/2, Sum3/2  "<Solar_Radiation_diffuse_surface>"
  Bus Selector/1 -> qp rad/1(Ta), Sum/1  "<Temperature_Ambient>"
  Bus Selector/2 -> qp rad/3(Tsky)  "<Temperature_Sky_Radiation>"
  Bus Selector/3 -> alfa/1  "<Wind_Speed>"
  surface of window/1 -> Bus Assignment2/2
  S_initialize/1 -> Bus Assignment2/1
  Bus Assignment2/1 -> "[S]"/1

== system carnotUIBK_bus/window/window_TF/lambda_window ==
  note: Heat conduction in a window (ONLY SURFACE LAYER CONNECTABLE)
  note: Timeconstant of window is calculated
      | in the mask initialization
  qdots1 : Inport
  qdots2 : Inport  Port=2
  Product1 : Product  InputSameDT=on  RndMeth=Zero  SaturateOnIntegerOverflow=on  OutDataTypeStr=Inherit: Same as first input
  Product6 : Product  InputSameDT=on  RndMeth=Zero  SaturateOnIntegerOverflow=on  OutDataTypeStr=Inherit: Same as first input
  R_win : Constant  Value=Rwin
  Sum1 : Sum  InputSameDT=on  SaturateOnIntegerOverflow=on  OutDataTypeStr=Inherit: Same as first input
  Sum3 : Sum  InputSameDT=on  SaturateOnIntegerOverflow=on  OutDataTypeStr=Inherit: Same as first input
  Transfer Fcn : TransferFcn  Denominator=[timeconst 1]
  Transfer Fcn1 : TransferFcn  Denominator=[timeconst 1]
  Ts1 : Outport  VectorParamsAs1DForOutWhenUnconnected=off
  Ts2 : Outport  Port=2  VectorParamsAs1DForOutWhenUnconnected=off
  wires:
  Transfer Fcn1/1 -> Ts2/1, Sum3/2
  Transfer Fcn/1 -> Ts1/1, Sum1/2
  qdots1/1 -> Product6/2
  qdots2/1 -> Product1/2
  Product6/1 -> Sum3/1
  Sum3/1 -> Transfer Fcn/1
  Product1/1 -> Sum1/1
  Sum1/1 -> Transfer Fcn1/1
  R_win/1 -> Product6/1, Product1/1  "R_win"
